simulink model "Q3"  (R2021a)
settings: Solver=VariableStepAuto  StartTime=0.0  StopTime=20  RelTol=1e-3
settings Model: Creator=hamed  LastModifiedBy=mg1121
settings SolverCC: AlgebraicLoopSolver=TrustRegion
settings DebuggingCC: SFMachineParentedDataDiag=warning

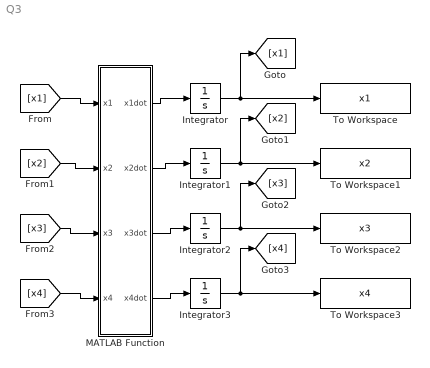
== system Q3 ==
  Integrator : Integrator  InitialCondition=1
  Integrator1 : Integrator  InitialCondition=2
  Integrator2 : Integrator
  Integrator3 : Integrator  InitialCondition=5
  MATLAB Function : MATLAB Function  TreatAsAtomicUnit=on
  To Workspace : ToWorkspace  VariableName=x1  SaveFormat=Timeseries  SampleTime=-1
  To Workspace1 : ToWorkspace  VariableName=x2  SaveFormat=Timeseries  SampleTime=-1
  To Workspace2 : ToWorkspace  VariableName=x3  SaveFormat=Timeseries  SampleTime=-1
  To Workspace3 : ToWorkspace  VariableName=x4  SaveFormat=Timeseries  SampleTime=-1
  wires:
  Integrator/1 -> [x1], To Workspace/1
  MATLAB Function/1(x1dot) -> Integrator/1
  [x1] -> MATLAB Function/1(x1)
  [x2] -> MATLAB Function/2(x2)
  [x3] -> MATLAB Function/3(x3)
  [x4] -> MATLAB Function/4(x4)
  MATLAB Function/2(x2dot) -> Integrator1/1
  Integrator1/1 -> [x2], To Workspace1/1
  MATLAB Function/3(x3dot) -> Integrator2/1
  Integrator2/1 -> [x3], To Workspace2/1
  MATLAB Function/4(x4dot) -> Integrator3/1
  Integrator3/1 -> [x4], To Workspace3/1

== matlab function Q3/MATLAB Function ==
  data: x1 input; x1dot output; x2 input; x2dot output; x3 input; x4 input; x3dot output; x4dot output

function [x1dot,x2dot,x3dot,x4dot] = fcn(x1,x2,x3,x4)

k=2;
x1dot = k*x1;
x2dot = k*(x1-x2);
x3dot = k*(x1-x3);
x4dot = k*(x2+x3-x4);
